simulink model "gm_pmsm_fpga_pcie_slrt"  (R2020b)
settings: Solver=FixedStepDiscrete  StartTime=0.0  StopTime=5  FixedStep=1e-5  RelTol=1e-3
PostLoadFcn:
  | try
  | cell = struct2cell(dir(fullfile(speedgoatroot_hdlb, 'hdlsrc', 'pwm', '*.vhd')));
  | addSourceFiles = strjoin(fullfile(cell(2,:),cell(1,:)), ';');
  | hdlset_param('pwm_example_hdlc/DUT PWM and CAP', 'IPCoreAdditionalFiles', addSourceFiles);
  | end
undefined symbols (not defined in the file): ee_sli_rtmsupport, FPGA, fsw, gcbh, IO334, J, Ld, Lq, N, PM, Pmax, pmsm_fpga_pcie, Tmax, Ts, Tsc
libraries: speedgoatlib_hdlCoder_IO3xx x19, fl_lib x10, nesl_utility x8, ee_lib x3, eeTransforms x2, quadrature_cpulib x1, slrealtimeutilitieslib x1, eePmsmCurrentController x1, eePmsmCurrentReferenceGen x1, eeVelocityController x1, eePwmGeneratorTwoLevel x1, pwm_cpulib x1
(part 2 of 2)

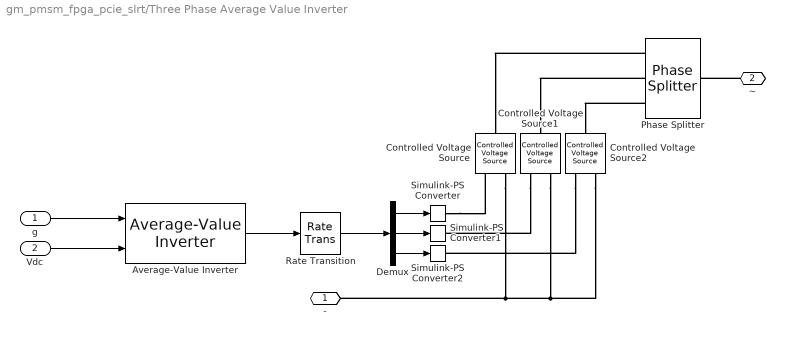
== system gm_pmsm_fpga_pcie_slrt/Three Phase Average Value Inverter ==
  g : Inport
  Vdc : Inport  Port=2
  Average-Value Inverter : mcbplantlib/Average-Value Inverter
  Controlled Voltage Source : fl_lib/Electrical/Electrical Sources/Controlled Voltage Source
  Controlled Voltage Source1 : fl_lib/Electrical/Electrical Sources/Controlled Voltage Source
  Controlled Voltage Source2 : fl_lib/Electrical/Electrical Sources/Controlled Voltage Source
  Demux : Demux  Outputs=3
  Phase Splitter : ee_lib/Connectors & References/Phase Splitter
      settings: SourceProductBaseCode=PS
  Rate Transition : RateTransition
  Simulink-PS Converter : nesl_utility/Simulink-PS Converter  PhysicalDomain=network_engine_domain  SubClassName=ps_input  LeftPortType=input  RightPortType=output  PseudoPeriodic=off  Frequencies=[]  NoiseDistribution=none  NoiseParameters=[]  Unit=1  AffineConversion=off  FilteringAndDerivatives=provide  SimscapeFilterOrder=1  InputFilterTimeConstant=0.001  UdotUserProvided=0
  Simulink-PS Converter1 : nesl_utility/Simulink-PS Converter  PhysicalDomain=network_engine_domain  SubClassName=ps_input  LeftPortType=input  RightPortType=output  PseudoPeriodic=off  Frequencies=[]  NoiseDistribution=none  NoiseParameters=[]  Unit=1  AffineConversion=off  FilteringAndDerivatives=provide  SimscapeFilterOrder=1  InputFilterTimeConstant=0.001  UdotUserProvided=0
  Simulink-PS Converter2 : nesl_utility/Simulink-PS Converter  PhysicalDomain=network_engine_domain  SubClassName=ps_input  LeftPortType=input  RightPortType=output  PseudoPeriodic=off  Frequencies=[]  NoiseDistribution=none  NoiseParameters=[]  Unit=1  AffineConversion=off  FilteringAndDerivatives=provide  SimscapeFilterOrder=1  InputFilterTimeConstant=0.001  UdotUserProvided=0
  - : PMIOPort  Tag=PMCPort  Side=Left
  ~ : PMIOPort  Tag=PMCPort  Port=2  Side=Right
  wires:
  Average-Value Inverter/1 -> Rate Transition/1
  Rate Transition/1 -> Demux/1
  g/1 -> Average-Value Inverter/1
  Demux/1 -> Simulink-PS Converter/1
  Demux/2 -> Simulink-PS Converter1/1
  Vdc/1 -> Average-Value Inverter/2
  Demux/3 -> Simulink-PS Converter2/1
  connections:
  Controlled Voltage Source1/RConn1 -- Simulink-PS Converter1/RConn1
  Phase Splitter/RConn2 -- Controlled Voltage Source1/LConn1
  Phase Splitter/RConn1 -- Controlled Voltage Source/LConn1
  Phase Splitter/RConn3 -- Controlled Voltage Source2/LConn1
  Controlled Voltage Source2/RConn1 -- Simulink-PS Converter2/RConn1
  Simulink-PS Converter/RConn1 -- Controlled Voltage Source/RConn1
  Controlled Voltage Source2/RConn2 -- Controlled Voltage Source1/RConn2 -- -/RConn1 -- Controlled Voltage Source/RConn2
  ~/RConn1 -- Phase Splitter/LConn1

== system gm_pmsm_fpga_pcie_slrt/FPGA/Packer ==
  unpacked : Inport
  pack : slrealtimeutilitieslib/Bit Packing  MaskBitPatterns={[0:15 16:31 32:47 ]}  MaskPackDataType=uint32  MaskPackDataSize=2
      settings: SourceProductBaseCode=XP
  sSpec : SignalSpecification  OutDataTypeStr=fixdt(1,16,0)
  upconvert : DataTypeConversion  OutDataTypeStr=uint16  ConvertRealWorld=Stored Integer (SI)  RndMeth=Zero
  packed : Outport
  wires:
  unpacked/1 -> sSpec/1
  sSpec/1 -> upconvert/1
  upconvert/1 -> pack/1
  pack/1 -> packed/1

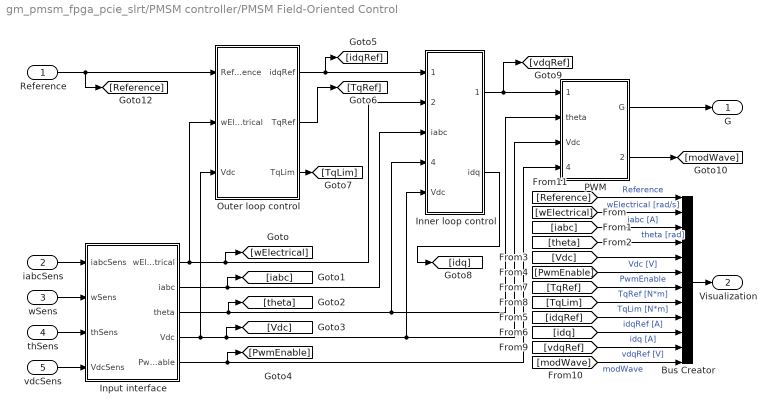
== system gm_pmsm_fpga_pcie_slrt/PMSM controller/PMSM Field-Oriented Control ==
  Reference : Inport  SampleTime=Tsc
  iabcSens : Inport  Port=2  SampleTime=Tsc
  wSens : Inport  Port=3  SampleTime=Tsc
  thSens : Inport  Port=4  SampleTime=Tsc
  vdcSens : Inport  Port=5  SampleTime=Tsc
  Bus Creator : BusCreator  Inputs=12
  Inner loop control : Subsystem
  Input interface : Subsystem
  Outer loop control : Subsystem
  PWM : Subsystem
  G : Outport  VectorParamsAs1DForOutWhenUnconnected=off
  Visualization : Outport  Port=2  VectorParamsAs1DForOutWhenUnconnected=off
  wires:
  Input interface/2(iabc) -> [iabc], Inner loop control/3(iabc)
  Input interface/3(theta) -> [theta], PWM/2(theta), Inner loop control/4(theta)
  Outer loop control/1(idqRef) -> [idqRef], Inner loop control/1(idq_ref)
  iabcSens/1 -> Input interface/1(iabcSens)
  wSens/1 -> Input interface/2(wSens)
  thSens/1 -> Input interface/3(thSens)
  vdcSens/1 -> Input interface/4(VdcSens)
  Reference/1 -> [Reference], Outer loop control/1(Reference)
  Input interface/4(Vdc) -> [Vdc], PWM/3(Vdc), Inner loop control/5(Vdc), Outer loop control/3(Vdc)
  Input interface/1(wElectrical) -> [wElectrical], Inner loop control/2(wElectrical), Outer loop control/2(wElectrical)
  Inner loop control/1(vdqRef) -> [vdqRef], PWM/1(vdqRef)
  Input interface/5(PwmEnable) -> [PwmEnable], PWM/4(PwmEnable)
  PWM/1(G) -> G/1
  Bus Creator/1 -> Visualization/1
  Outer loop control/2(TqRef) -> [TqRef]
  Outer loop control/3(TqLim) -> [TqLim]
  Inner loop control/2(idq) -> [idq]
  PWM/2(ModWave) -> [modWave]
  [Reference] -> Bus Creator/1  "Reference"
  [wElectrical] -> Bus Creator/2  "wElectrical [rad/s]"
  [iabc] -> Bus Creator/3  "iabc [A]"
  [theta] -> Bus Creator/4  "theta [rad]"
  [Vdc] -> Bus Creator/5  "Vdc [V]"
  [PwmEnable] -> Bus Creator/6  "PwmEnable"
  [TqRef] -> Bus Creator/7  "TqRef [N*m]"
  [TqLim] -> Bus Creator/8  "TqLim [N*m]"
  [idqRef] -> Bus Creator/9  "idqRef [A]"
  [idq] -> Bus Creator/10  "idq [A]"
  [vdqRef] -> Bus Creator/11  "vdqRef [V]"
  [modWave] -> Bus Creator/12  "modWave"

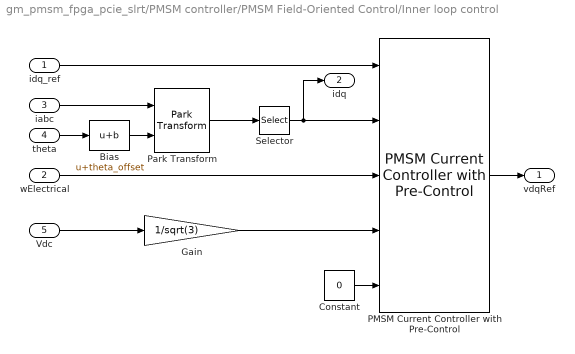
== system gm_pmsm_fpga_pcie_slrt/PMSM controller/PMSM Field-Oriented Control/Inner loop control ==
  idq_ref : Inport
  wElectrical : Inport  Port=2
  iabc : Inport  Port=3
  theta : Inport  Port=4
  Vdc : Inport  Port=5
  Bias : Bias  Bias=theta_offset
  Constant : Constant  Value=0  SampleTime=-1
  Gain : Gain  Gain=1/sqrt(3)
  PMSM Current Controller with Pre-Control : eePmsmCurrentController/PMSM Current Controller with Pre-Control  Kp_id=Kp_id  Ki_id=Ki_id  Kaw_id=Kaw_id  Kp_iq=Kp_iq  Ki_iq=Ki_iq  Kaw_iq=Kaw_iq  Ts=Tsc  Tsd=0.001  AxisPrio=Q-axis  ActZC=off  ActFF=on  idVect=idVect  iqVect=iqVect  LdMatrix=LdMatrix  LqMatrix=LqMatrix  psimMatrix=psimMatrix
      settings: SourceProductBaseCode=PS
  Park Transform : eeTransforms/Park Transform  AxisAlignment=Q-axis  PowerInvariant=off
  Selector : Selector  InputPortWidth=3  IndexOptions=Index vector (dialog)  Indices=[1 2]  OutputSizes=1
  vdqRef : Outport  VectorParamsAs1DForOutWhenUnconnected=off
  idq : Outport  Port=2  VectorParamsAs1DForOutWhenUnconnected=off
  wires:
  Constant/1 -> PMSM Current Controller with Pre-Control/5
  Selector/1 -> PMSM Current Controller with Pre-Control/2, idq/1
  Gain/1 -> PMSM Current Controller with Pre-Control/4
  Park Transform/1 -> Selector/1
  idq_ref/1 -> PMSM Current Controller with Pre-Control/1
  iabc/1 -> Park Transform/1
  theta/1 -> Bias/1
  wElectrical/1 -> PMSM Current Controller with Pre-Control/3
  Vdc/1 -> Gain/1
  PMSM Current Controller with Pre-Control/1 -> vdqRef/1
  Bias/1 -> Park Transform/2

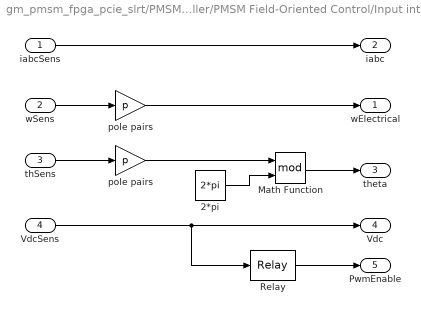
== system gm_pmsm_fpga_pcie_slrt/PMSM controller/PMSM Field-Oriented Control/Input interface ==
  iabcSens : Inport
  wSens : Inport  Port=2
  thSens : Inport  Port=3
  VdcSens : Inport  Port=4
  2*pi : Constant  Value=2*pi  SampleTime=Tsc
  Math Function : Math  Operator=mod  SignedPower=on  SaturateOnIntegerOverflow=on
  Relay : Relay  OnSwitchValue=Vdc_on  OffSwitchValue=0.5*Vdc_on
  pole pairs : Gain  Gain=p
  "pole pairs " : Gain  Gain=p
  wElectrical : Outport  VectorParamsAs1DForOutWhenUnconnected=off
  iabc : Outport  Port=2  VectorParamsAs1DForOutWhenUnconnected=off
  theta : Outport  Port=3  VectorParamsAs1DForOutWhenUnconnected=off
  Vdc : Outport  Port=4  VectorParamsAs1DForOutWhenUnconnected=off
  PwmEnable : Outport  Port=5  VectorParamsAs1DForOutWhenUnconnected=off
  wires:
  pole pairs/1 -> wElectrical/1
  thSens/1 -> "pole pairs "/1
  wSens/1 -> pole pairs/1
  iabcSens/1 -> iabc/1
  "pole pairs "/1 -> Math Function/1
  2*pi/1 -> Math Function/2
  Math Function/1 -> theta/1
  Relay/1 -> PwmEnable/1
  VdcSens/1 -> Relay/1, Vdc/1

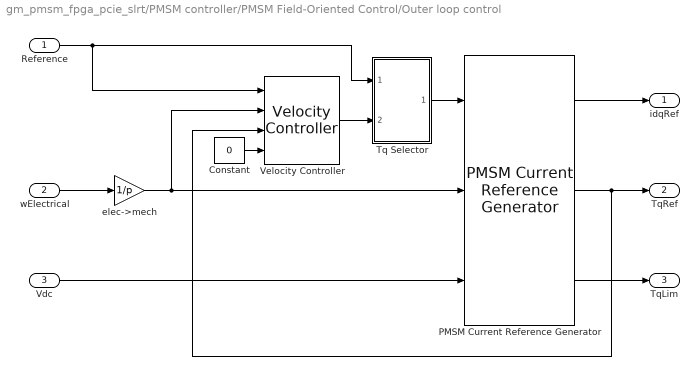
== system gm_pmsm_fpga_pcie_slrt/PMSM controller/PMSM Field-Oriented Control/Outer loop control ==
  Reference : Inport
  wElectrical : Inport  Port=2
  Vdc : Inport  Port=3
  Constant : Constant  Value=0  SampleTime=-1
  PMSM Current Reference Generator : eePmsmCurrentReferenceGen/PMSM Current Reference Generator  Vnom=Vnom  Pmax=Pmax  Tmax=Tmax  Ts=Tsc  RefType=Zero d-axis control  rpmVec=rpmVec  TqVec=TqVec  VdcVec=VdcVec  PWMMode=SPWM: sinusoidal PWM  ModFactor=ModFactor  idMatrix=idMatrix  iqMatrix=iqMatrix  p=p  psim=psim  Ld=Ld  Lq=Lq  Rs=Rs  RefExpEnable=0
      settings: SourceProductBaseCode=PS
  Tq Selector : Subsystem
  Velocity Controller : eeVelocityController/Velocity Controller  CtrlType=PI control  Kp_w=Kp_w  Ki_w=Ki_w  Kv_w=Kv_w  Kaw_w=Kaw_w  Ts=Tsc  Tsd=0.001  ActZC=off
      settings: SourceProductBaseCode=PS
  elec->mech : Gain  Gain=1/p
  idqRef : Outport  VectorParamsAs1DForOutWhenUnconnected=off
  TqRef : Outport  Port=2  VectorParamsAs1DForOutWhenUnconnected=off
  TqLim : Outport  Port=3  VectorParamsAs1DForOutWhenUnconnected=off
  wires:
  Reference/1 -> Velocity Controller/1, Tq Selector/1(Reference)
  wElectrical/1 -> elec->mech/1
  Vdc/1 -> PMSM Current Reference Generator/3
  PMSM Current Reference Generator/1 -> idqRef/1
  PMSM Current Reference Generator/2 -> Velocity Controller/3, TqRef/1
  PMSM Current Reference Generator/3 -> TqLim/1
  elec->mech/1 -> PMSM Current Reference Generator/2, Velocity Controller/2
  Constant/1 -> Velocity Controller/4
  Tq Selector/1(TqRef) -> PMSM Current Reference Generator/1
  Velocity Controller/1 -> Tq Selector/2(TqRefUnsat)

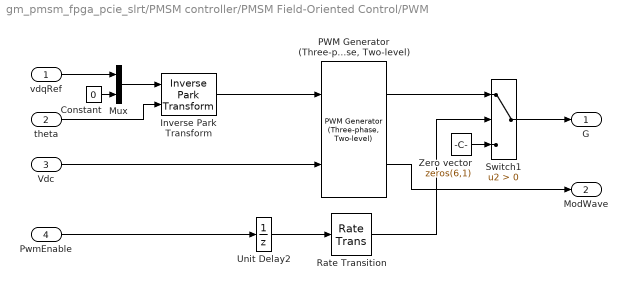
== system gm_pmsm_fpga_pcie_slrt/PMSM controller/PMSM Field-Oriented Control/PWM ==
  vdqRef : Inport
  theta : Inport  Port=2
  Vdc : Inport  Port=3
  PwmEnable : Inport  Port=4
  Constant : Constant  Value=0  SampleTime=Tsc
  Inverse Park Transform : eeTransforms/Inverse Park Transform  AxisAlignment=Q-axis  PowerInvariant=off
  Mux : Mux  Inputs=2
  "PWM Generator (Three-phase, Two-level)" : eePwmGeneratorTwoLevel/PWM Generator (Three-phase, Two-level)  PWMMode=Continuous PWM (CPWM)  CPWMMode=SPWM: sinusoidal PWM  DPWMMode=60 DPWM: 60 degree discontinuous PWM  fsw=fsw  Ts=Ts
      settings: SourceProductBaseCode=PS
  Rate Transition : RateTransition
  Switch1 : Switch  Criteria=u2 > Threshold
  Unit Delay2 : UnitDelay  SampleTime=Tsc  HasFrameUpgradeWarning=on
  Zero vector : Constant  Value=zeros(6,1)  SampleTime=Ts
  G : Outport  VectorParamsAs1DForOutWhenUnconnected=off
  ModWave : Outport  Port=2  SampleTime=Tsc  VectorParamsAs1DForOutWhenUnconnected=off
  wires:
  theta/1 -> Inverse Park Transform/2
  vdqRef/1 -> Mux/1
  Mux/1 -> Inverse Park Transform/1
  Constant/1 -> Mux/2
  "PWM Generator (Three-phase, Two-level)"/2 -> ModWave/1
  "PWM Generator (Three-phase, Two-level)"/1 -> Switch1/1
  PwmEnable/1 -> Unit Delay2/1
  Zero vector/1 -> Switch1/3
  Switch1/1 -> G/1
  Inverse Park Transform/1 -> "PWM Generator (Three-phase, Two-level)"/1
  Vdc/1 -> "PWM Generator (Three-phase, Two-level)"/2
  Unit Delay2/1 -> Rate Transition/1
  Rate Transition/1 -> Switch1/2

== system gm_pmsm_fpga_pcie_slrt/PMSM controller/PMSM Field-Oriented Control/Outer loop control/Tq Selector ==
  Reference : Inport
  TqRefUnsat : Inport  Port=2
  Constant : Constant  Value=CtrlMode  SampleTime=Tsc
  Switch : Switch  Criteria=u2 > Threshold  Threshold=1.5
  TqRef : Outport  VectorParamsAs1DForOutWhenUnconnected=off
  wires:
  Reference/1 -> Switch/1
  TqRefUnsat/1 -> Switch/3
  Constant/1 -> Switch/2
  Switch/1 -> TqRef/1
